simulink model "benchmark_model"  (R2021a)
settings: Solver=ode1  StartTime=0.0  StopTime=Tend  FixedStep=0.0001  MaxStep=0.1  MinStep=0.0001  AbsTol=0.01  EnableMultiTasking=on
undefined symbols (not defined in the file): A1, A2, AL, AM0, AREA, BORE, C_EGR, c_f, c_T, CAIR, cCO, cCO2, cH2, cH2O, cHC, cN2, CO, CO2, cO2, DEN0, DiscIntNeverNeededParam, EGR_dia, EGR_sk, EX_AREA, EX_M_AR, EXO, FD0, FOM, FR0, FR_C1, FR_C2, FR_C3, FR_C4, FR_C5, H2, H2O, HC, INC, INO, KET, Kex, Kh, MAS0, MCh, MHC, MN2, MO2, MOLcylT, N2, O2, PR0, R150, Rabs, SPEC, TBORE, Th_HC, Th_knock, THEX, THIN, TM0 ... (+9)
libraries: pid_lib x1
(part 2 of 6)

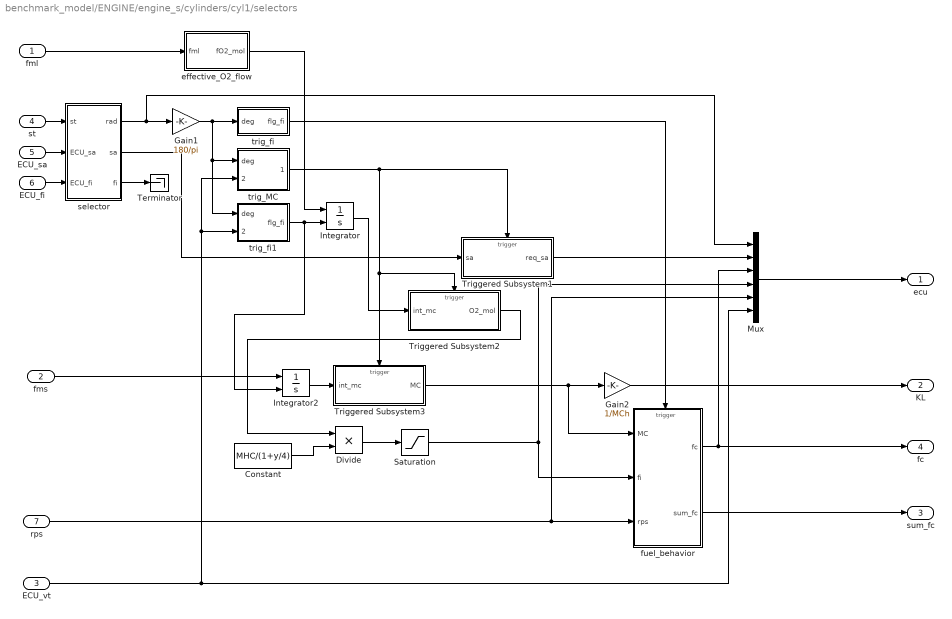
== system benchmark_model/ENGINE/engine_s/cylinders/cyl1/selectors ==
  fml : Inport
  fms : Inport  Port=2
  ECU_vt : Inport  Port=3
  st : Inport  Port=4
  ECU_sa : Inport  Port=5
  ECU_fi : Inport  Port=6
  rps : Inport  Port=7
  Constant : Constant  Value=MHC/(1+y/4)
  Divide : Product
  Gain1 : Gain  Gain=180/pi
  Gain2 : Gain  Gain=1/MCh
  Integrator : Integrator  ExternalReset=rising
  Integrator2 : Integrator  ExternalReset=rising
  Mux : Mux  Inputs=6
  Saturation : Saturate  UpperLimit=inf  LowerLimit=0
  Terminator : Terminator
  Triggered Subsystem1 : Subsystem  TreatAsAtomicUnit=on
  Triggered Subsystem2 : Subsystem  TreatAsAtomicUnit=on
  Triggered Subsystem3 : Subsystem  TreatAsAtomicUnit=on
  effective_O2_flow : Subsystem
  fuel_behavior : Subsystem  TreatAsAtomicUnit=on
  selector : Subsystem
  trig_MC : Subsystem
  trig_fi : Subsystem
  trig_fi1 : Subsystem
  ecu : Outport
  KL : Outport  Port=2
  sum_fc : Outport  Port=3
  fc : Outport  Port=4
  wires:
  Triggered Subsystem2/1(O2_mol) -> Divide/1
  Gain1/1 -> trig_fi/1(deg), trig_fi1/1(deg), trig_MC/1(deg)
  ECU_fi/1 -> selector/3(ECU_fi)
  ECU_sa/1 -> selector/2(ECU_sa)
  st/1 -> selector/1(st)
  trig_MC/1(flg_inc) -> Triggered Subsystem3/Trigger, Triggered Subsystem2/Trigger, Triggered Subsystem1/Trigger
  rps/1 -> Mux/5, fuel_behavior/3(rps)
  selector/1(rad) -> Gain1/1, Mux/1
  Mux/1 -> ecu/1
  trig_fi/1(flg_fi) -> fuel_behavior/Trigger
  selector/2(sa) -> Triggered Subsystem1/1(sa)
  Triggered Subsystem1/1(req_sa) -> Mux/2
  trig_fi1/1(flg_fi) -> Integrator/2, Integrator2/2
  Integrator/1 -> Triggered Subsystem2/1(int_mc)
  fuel_behavior/1(fc) -> fc/1, Mux/3
  selector/3(fi) -> Terminator/1
  Gain2/1 -> KL/1
  Divide/1 -> Saturation/1
  fml/1 -> effective_O2_flow/1(fml)
  effective_O2_flow/1(fO2_mol) -> Integrator/1
  Constant/1 -> Divide/2
  Saturation/1 -> fuel_behavior/2(fi), Mux/4
  Integrator2/1 -> Triggered Subsystem3/1(int_mc)
  Triggered Subsystem3/1(MC) -> Gain2/1, fuel_behavior/1(MC)
  fms/1 -> Integrator2/1
  ECU_vt/1 -> trig_MC/2(ECU_vvt), trig_fi1/2(ECU_vvt), Mux/6
  fuel_behavior/2(sum_fc) -> sum_fc/1

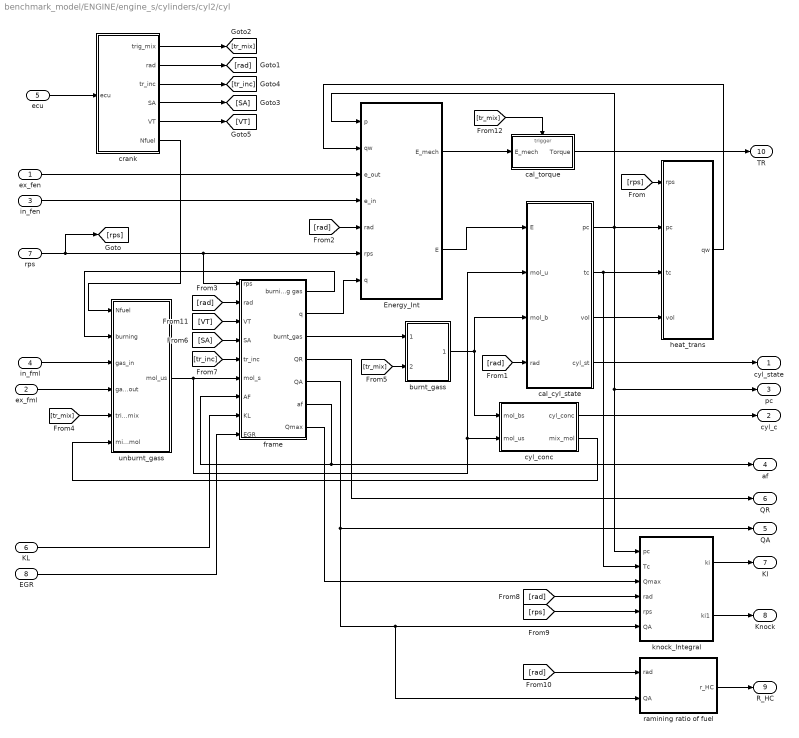
== system benchmark_model/ENGINE/engine_s/cylinders/cyl2/cyl ==
  ex_fen : Inport
  ex_fml : Inport  Port=2
  in_fen : Inport  Port=3
  in_fml : Inport  Port=4
  ecu : Inport  Port=5
  KL : Inport  Port=6
  rps : Inport  Port=7
  EGR : Inport  Port=8
  Energy_Int : Subsystem
  burnt_gass : Subsystem
  cal_cyl_state : Subsystem
  cal_torque : Subsystem
  crank : Subsystem
  cyl_conc : Subsystem
  frame : Subsystem
  heat_trans : Subsystem
  knock_Integral : Subsystem
  ramining ratio of fuel : Subsystem
  unburnt_gass : Subsystem
  cyl_state : Outport  InitialOutput=0
  cyl_c : Outport  Port=2  InitialOutput=0
  pc : Outport  Port=3  InitialOutput=0
  af : Outport  Port=4  InitialOutput=0
  QA : Outport  Port=5  InitialOutput=0
  QR : Outport  Port=6  InitialOutput=0
  KI : Outport  Port=7  InitialOutput=0
  Knock : Outport  Port=8  InitialOutput=0
  R_HC : Outport  Port=9  InitialOutput=0
  TR : Outport  Port=10  InitialOutput=0
  wires:
  [tr_mix] -> cal_torque/Trigger
  cal_torque/1(Torque) -> TR/1
  Energy_Int/1(E_mech) -> cal_torque/1(E_mech)
  crank/5(VT) -> [VT]
  [VT] -> frame/3(VT)
  frame/7(Qmax) -> knock_Integral/3(Qmax)
  ramining ratio of fuel/1(r_HC) -> R_HC/1
  [rad] -> ramining ratio of fuel/1(rad)
  knock_Integral/2(ki1) -> Knock/1
  [rps] -> knock_Integral/5(rps)
  frame/5(QA) -> knock_Integral/6(QA), ramining ratio of fuel/2(QA), QA/1
  [rad] -> knock_Integral/4(rad)
  EGR/1 -> frame/9(EGR)
  knock_Integral/1(ki) -> KI/1
  frame/4(QR) -> QR/1
  KL/1 -> frame/8(KL)
  [SA] -> frame/4(SA)
  crank/4(SA) -> [SA]
  Energy_Int/2(E) -> cal_cyl_state/1(E)
  cal_cyl_state/2(tc) -> heat_trans/3(tc), knock_Integral/2(Tc)
  cal_cyl_state/3(vol) -> heat_trans/4(vol)
  cal_cyl_state/4(cyl_st) -> cyl_state/1
  [rad] -> cal_cyl_state/4(rad)
  cal_cyl_state/1(pc) -> knock_Integral/1(pc), pc/1, Energy_Int/1(p), heat_trans/2(pc)
  crank/3(tr_inc) -> [tr_inc]
  cyl_conc/2(mix_mol) -> unburnt_gass/6(mix_mol)
  [tr_inc] -> frame/5(tr_inc)
  crank/6(Nfuel) -> unburnt_gass/1(Nfuel)
  frame/6(af) -> frame/7(AF), af/1
  crank/2(rad) -> [rad]
  [tr_mix] -> burnt_gass/2(tr_mix)
  [tr_mix] -> unburnt_gass/5(trig_mix)
  crank/1(trig_mix) -> [tr_mix]
  frame/1(burning gas) -> unburnt_gass/2(burning)
  ex_fml/1 -> unburnt_gass/4(gas_out)
  in_fen/1 -> Energy_Int/4(e_in)
  ex_fen/1 -> Energy_Int/3(e_out)
  [rad] -> frame/2(rad)
  [rad] -> Energy_Int/5(rad)
  ecu/1 -> crank/1(ecu)
  [rps] -> heat_trans/1(rps)
  cyl_conc/1(cyl_conc) -> cyl_c/1
  burnt_gass/1(mol_bs) -> cyl_conc/1(mol_bs), cal_cyl_state/3(mol_b)
  in_fml/1 -> unburnt_gass/3(gas_in)
  rps/1 -> Energy_Int/6(rps), frame/1(rps), [rps]
  unburnt_gass/1(mol_us) -> frame/6(mol_s), cal_cyl_state/2(mol_u), cyl_conc/2(mol_us)
  frame/3(burnt_gas) -> burnt_gass/1(gas_in)
  frame/2(q) -> Energy_Int/7(q)
  heat_trans/1(qw) -> Energy_Int/2(qw)

== system benchmark_model/ENGINE/engine_s/cylinders/cyl2/ex_valve ==
  d_st : Inport
  d_c : Inport  Port=2
  ecu : Inport  Port=3
  u_st : Inport  Port=4  PortDimensions=4
  u_c : Inport  Port=5
  Constant : Constant  Value=WOM
  Constant1 : Constant  Value=4*pi
  Gain : Gain  Gain=180/pi
  Lookup Table1 : Lookup  InputValues=THEX  Table=VAREX
  Math Function : Math  Operator=mod  SignedPower=on  SaturateOnIntegerOverflow=on
  Selector : Selector  InputPortWidth=6  IndexOptions=Index vector (dialog)  Indices=1  OutputSizes=[(-2)]
  cal_flow : MATLAB Function  TreatAsAtomicUnit=on
  fen : Outport  PortDimensions=1
  fml : Outport  Port=2  PortDimensions=7
  wires:
  Constant1/1 -> Math Function/2
  Selector/1 -> Math Function/1
  Math Function/1 -> Gain/1
  Gain/1 -> Lookup Table1/1
  Constant/1 -> cal_flow/6(WOM)
  cal_flow/2(fml) -> fml/1
  d_c/1 -> cal_flow/5(c_out)
  d_st/1 -> cal_flow/4(outlet)
  u_c/1 -> cal_flow/3(c_in)
  u_st/1 -> cal_flow/2(inlet)
  Lookup Table1/1 -> cal_flow/1(area)
  cal_flow/1(fen) -> fen/1
  ecu/1 -> Selector/1

== system benchmark_model/ENGINE/engine_s/cylinders/cyl2/in_valve ==
  d_c : Inport
  d_st : Inport  Port=2
  ecu : Inport  Port=3
  in_vt : Inport  Port=4
  u_st : Inport  Port=5
  u_c : Inport  Port=6
  Add : Sum  Inputs=-+
  Constant : Constant  Value=WOM
  Gain : Gain  Gain=180/pi
  Lookup Table : Lookup  InputValues=THIN  Table=VARIN
  Selector1 : Selector  InputPortWidth=6  IndexOptions=Index vector (dialog)  Indices=1  OutputSizes=[(-2)]
  cal_flow : MATLAB Function  TreatAsAtomicUnit=on
  fen : Outport  PortDimensions=1
  fml : Outport  Port=2  PortDimensions=7
  fms : Outport  Port=3  PortDimensions=1
  wires:
  Add/1 -> Gain/1
  Selector1/1 -> Add/2
  in_vt/1 -> Add/1
  Constant/1 -> cal_flow/6(WOM)
  cal_flow/3(fms) -> fms/1
  cal_flow/2(fml) -> fml/1
  d_c/1 -> cal_flow/5(c_out)
  u_c/1 -> cal_flow/3(c_in)
  cal_flow/1(fen) -> fen/1
  d_st/1 -> cal_flow/4(outlet)
  Lookup Table/1 -> cal_flow/1(area)
  u_st/1 -> cal_flow/2(inlet)
  ecu/1 -> Selector1/1
  Gain/1 -> Lookup Table/1

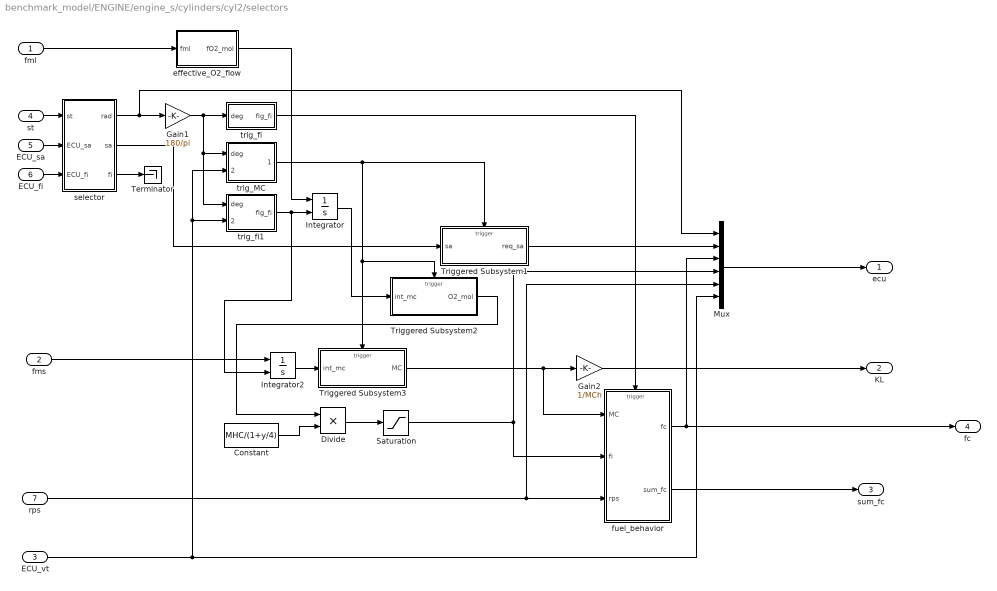
== system benchmark_model/ENGINE/engine_s/cylinders/cyl2/selectors ==
  fml : Inport
  fms : Inport  Port=2
  ECU_vt : Inport  Port=3
  st : Inport  Port=4
  ECU_sa : Inport  Port=5
  ECU_fi : Inport  Port=6
  rps : Inport  Port=7
  Constant : Constant  Value=MHC/(1+y/4)
  Divide : Product
  Gain1 : Gain  Gain=180/pi
  Gain2 : Gain  Gain=1/MCh
  Integrator : Integrator  ExternalReset=rising
  Integrator2 : Integrator  ExternalReset=rising
  Mux : Mux  Inputs=6
  Saturation : Saturate  UpperLimit=inf  LowerLimit=0
  Terminator : Terminator
  Triggered Subsystem1 : Subsystem  TreatAsAtomicUnit=on
  Triggered Subsystem2 : Subsystem  TreatAsAtomicUnit=on
  Triggered Subsystem3 : Subsystem  TreatAsAtomicUnit=on
  effective_O2_flow : Subsystem
  fuel_behavior : Subsystem  TreatAsAtomicUnit=on
  selector : Subsystem
  trig_MC : Subsystem
  trig_fi : Subsystem
  trig_fi1 : Subsystem
  ecu : Outport
  KL : Outport  Port=2
  sum_fc : Outport  Port=3
  fc : Outport  Port=4
  wires:
  fuel_behavior/2(sum_fc) -> sum_fc/1
  ECU_vt/1 -> Mux/6, trig_fi1/2(ECU_vvt), trig_MC/2(ECU_vvt)
  fms/1 -> Integrator2/1
  Triggered Subsystem3/1(MC) -> fuel_behavior/1(MC), Gain2/1
  Integrator2/1 -> Triggered Subsystem3/1(int_mc)
  Saturation/1 -> Mux/4, fuel_behavior/2(fi)
  Constant/1 -> Divide/2
  effective_O2_flow/1(fO2_mol) -> Integrator/1
  fml/1 -> effective_O2_flow/1(fml)
  Divide/1 -> Saturation/1
  Gain2/1 -> KL/1
  selector/3(fi) -> Terminator/1
  Integrator/1 -> Triggered Subsystem2/1(int_mc)
  trig_fi1/1(flg_fi) -> Integrator2/2, Integrator/2
  Triggered Subsystem1/1(req_sa) -> Mux/2
  selector/2(sa) -> Triggered Subsystem1/1(sa)
  trig_fi/1(flg_fi) -> fuel_behavior/Trigger
  Mux/1 -> ecu/1
  selector/1(rad) -> Mux/1, Gain1/1
  rps/1 -> fuel_behavior/3(rps), Mux/5
  trig_MC/1(flg_inc) -> Triggered Subsystem1/Trigger, Triggered Subsystem2/Trigger, Triggered Subsystem3/Trigger
  st/1 -> selector/1(st)
  ECU_sa/1 -> selector/2(ECU_sa)
  ECU_fi/1 -> selector/3(ECU_fi)
  Gain1/1 -> trig_MC/1(deg), trig_fi1/1(deg), trig_fi/1(deg)
  Triggered Subsystem2/1(O2_mol) -> Divide/1
  fuel_behavior/1(fc) -> fc/1, Mux/3

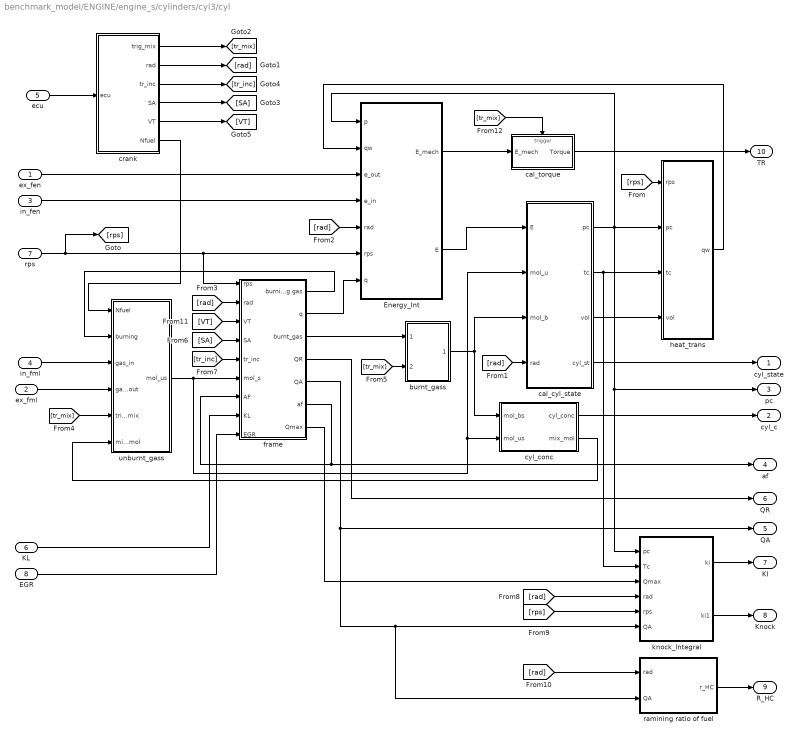
== system benchmark_model/ENGINE/engine_s/cylinders/cyl3/cyl ==
  ex_fen : Inport
  ex_fml : Inport  Port=2
  in_fen : Inport  Port=3
  in_fml : Inport  Port=4
  ecu : Inport  Port=5
  KL : Inport  Port=6
  rps : Inport  Port=7
  EGR : Inport  Port=8
  Energy_Int : Subsystem
  burnt_gass : Subsystem
  cal_cyl_state : Subsystem
  cal_torque : Subsystem
  crank : Subsystem
  cyl_conc : Subsystem
  frame : Subsystem
  heat_trans : Subsystem
  knock_Integral : Subsystem
  ramining ratio of fuel : Subsystem
  unburnt_gass : Subsystem
  cyl_state : Outport  InitialOutput=0
  cyl_c : Outport  Port=2  InitialOutput=0
  pc : Outport  Port=3  InitialOutput=0
  af : Outport  Port=4  InitialOutput=0
  QA : Outport  Port=5  InitialOutput=0
  QR : Outport  Port=6  InitialOutput=0
  KI : Outport  Port=7  InitialOutput=0
  Knock : Outport  Port=8  InitialOutput=0
  R_HC : Outport  Port=9  InitialOutput=0
  TR : Outport  Port=10  InitialOutput=0
  wires:
  heat_trans/1(qw) -> Energy_Int/2(qw)
  frame/2(q) -> Energy_Int/7(q)
  frame/3(burnt_gas) -> burnt_gass/1(gas_in)
  unburnt_gass/1(mol_us) -> cyl_conc/2(mol_us), cal_cyl_state/2(mol_u), frame/6(mol_s)
  rps/1 -> [rps], frame/1(rps), Energy_Int/6(rps)
  in_fml/1 -> unburnt_gass/3(gas_in)
  burnt_gass/1(mol_bs) -> cal_cyl_state/3(mol_b), cyl_conc/1(mol_bs)
  cyl_conc/1(cyl_conc) -> cyl_c/1
  [rps] -> heat_trans/1(rps)
  ecu/1 -> crank/1(ecu)
  [rad] -> Energy_Int/5(rad)
  [rad] -> frame/2(rad)
  ex_fen/1 -> Energy_Int/3(e_out)
  in_fen/1 -> Energy_Int/4(e_in)
  ex_fml/1 -> unburnt_gass/4(gas_out)
  frame/1(burning gas) -> unburnt_gass/2(burning)
  crank/1(trig_mix) -> [tr_mix]
  [tr_mix] -> unburnt_gass/5(trig_mix)
  [tr_mix] -> burnt_gass/2(tr_mix)
  crank/2(rad) -> [rad]
  frame/6(af) -> af/1, frame/7(AF)
  crank/6(Nfuel) -> unburnt_gass/1(Nfuel)
  [tr_inc] -> frame/5(tr_inc)
  cyl_conc/2(mix_mol) -> unburnt_gass/6(mix_mol)
  crank/3(tr_inc) -> [tr_inc]
  cal_cyl_state/1(pc) -> heat_trans/2(pc), Energy_Int/1(p), pc/1, knock_Integral/1(pc)
  [rad] -> cal_cyl_state/4(rad)
  cal_cyl_state/4(cyl_st) -> cyl_state/1
  cal_cyl_state/3(vol) -> heat_trans/4(vol)
  cal_cyl_state/2(tc) -> knock_Integral/2(Tc), heat_trans/3(tc)
  Energy_Int/2(E) -> cal_cyl_state/1(E)
  crank/4(SA) -> [SA]
  [SA] -> frame/4(SA)
  KL/1 -> frame/8(KL)
  frame/4(QR) -> QR/1
  knock_Integral/1(ki) -> KI/1
  EGR/1 -> frame/9(EGR)
  [rad] -> knock_Integral/4(rad)
  frame/5(QA) -> QA/1, ramining ratio of fuel/2(QA), knock_Integral/6(QA)
  [rps] -> knock_Integral/5(rps)
  knock_Integral/2(ki1) -> Knock/1
  [rad] -> ramining ratio of fuel/1(rad)
  ramining ratio of fuel/1(r_HC) -> R_HC/1
  frame/7(Qmax) -> knock_Integral/3(Qmax)
  [VT] -> frame/3(VT)
  crank/5(VT) -> [VT]
  Energy_Int/1(E_mech) -> cal_torque/1(E_mech)
  cal_torque/1(Torque) -> TR/1
  [tr_mix] -> cal_torque/Trigger

== system benchmark_model/ENGINE/engine_s/cylinders/cyl3/ex_valve ==
  d_st : Inport
  d_c : Inport  Port=2
  ecu : Inport  Port=3
  u_st : Inport  Port=4  PortDimensions=4
  u_c : Inport  Port=5
  Constant : Constant  Value=WOM
  Constant1 : Constant  Value=4*pi
  Gain : Gain  Gain=180/pi
  Lookup Table1 : Lookup  InputValues=THEX  Table=VAREX
  Math Function : Math  Operator=mod  SignedPower=on  SaturateOnIntegerOverflow=on
  Selector : Selector  InputPortWidth=6  IndexOptions=Index vector (dialog)  Indices=1  OutputSizes=[(-2)]
  cal_flow : MATLAB Function  TreatAsAtomicUnit=on
  fen : Outport  PortDimensions=1
  fml : Outport  Port=2  PortDimensions=7
  wires:
  ecu/1 -> Selector/1
  cal_flow/1(fen) -> fen/1
  Lookup Table1/1 -> cal_flow/1(area)
  u_st/1 -> cal_flow/2(inlet)
  u_c/1 -> cal_flow/3(c_in)
  d_st/1 -> cal_flow/4(outlet)
  d_c/1 -> cal_flow/5(c_out)
  cal_flow/2(fml) -> fml/1
  Constant/1 -> cal_flow/6(WOM)
  Gain/1 -> Lookup Table1/1
  Math Function/1 -> Gain/1
  Selector/1 -> Math Function/1
  Constant1/1 -> Math Function/2

== system benchmark_model/ENGINE/engine_s/cylinders/cyl3/in_valve ==
  d_c : Inport
  d_st : Inport  Port=2
  ecu : Inport  Port=3
  in_vt : Inport  Port=4
  u_st : Inport  Port=5
  u_c : Inport  Port=6
  Add : Sum  Inputs=-+
  Constant : Constant  Value=WOM
  Gain : Gain  Gain=180/pi
  Lookup Table : Lookup  InputValues=THIN  Table=VARIN
  Selector1 : Selector  InputPortWidth=6  IndexOptions=Index vector (dialog)  Indices=1  OutputSizes=[(-2)]
  cal_flow : MATLAB Function  TreatAsAtomicUnit=on
  fen : Outport  PortDimensions=1
  fml : Outport  Port=2  PortDimensions=7
  fms : Outport  Port=3  PortDimensions=1
  wires:
  Gain/1 -> Lookup Table/1
  ecu/1 -> Selector1/1
  u_st/1 -> cal_flow/2(inlet)
  Lookup Table/1 -> cal_flow/1(area)
  d_st/1 -> cal_flow/4(outlet)
  cal_flow/1(fen) -> fen/1
  u_c/1 -> cal_flow/3(c_in)
  d_c/1 -> cal_flow/5(c_out)
  cal_flow/2(fml) -> fml/1
  cal_flow/3(fms) -> fms/1
  Constant/1 -> cal_flow/6(WOM)
  in_vt/1 -> Add/1
  Selector1/1 -> Add/2
  Add/1 -> Gain/1

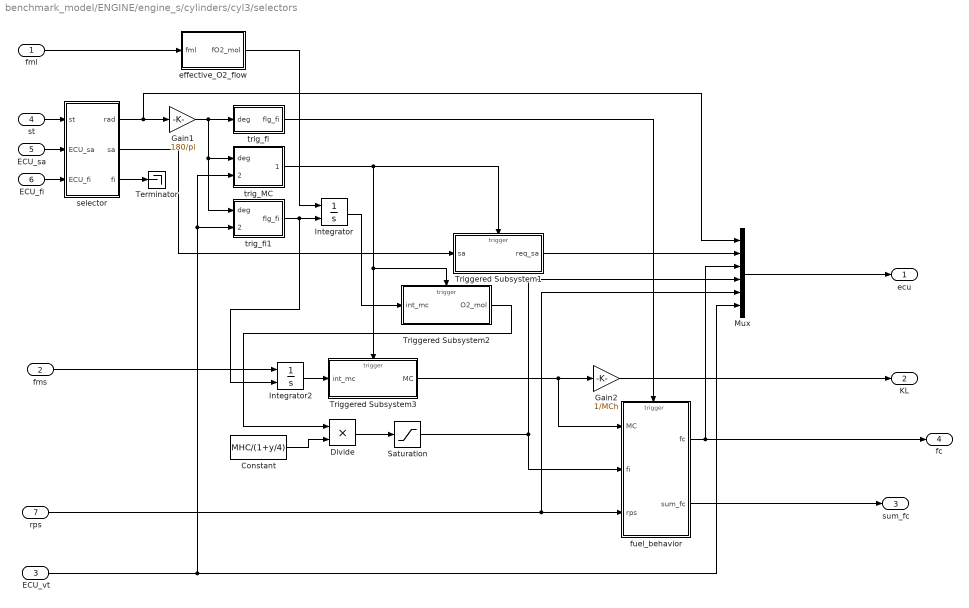
== system benchmark_model/ENGINE/engine_s/cylinders/cyl3/selectors ==
  fml : Inport
  fms : Inport  Port=2
  ECU_vt : Inport  Port=3
  st : Inport  Port=4
  ECU_sa : Inport  Port=5
  ECU_fi : Inport  Port=6
  rps : Inport  Port=7
  Constant : Constant  Value=MHC/(1+y/4)
  Divide : Product
  Gain1 : Gain  Gain=180/pi
  Gain2 : Gain  Gain=1/MCh
  Integrator : Integrator  ExternalReset=rising
  Integrator2 : Integrator  ExternalReset=rising
  Mux : Mux  Inputs=6
  Saturation : Saturate  UpperLimit=inf  LowerLimit=0
  Terminator : Terminator
  Triggered Subsystem1 : Subsystem  TreatAsAtomicUnit=on
  Triggered Subsystem2 : Subsystem  TreatAsAtomicUnit=on
  Triggered Subsystem3 : Subsystem  TreatAsAtomicUnit=on
  effective_O2_flow : Subsystem
  fuel_behavior : Subsystem  TreatAsAtomicUnit=on
  selector : Subsystem
  trig_MC : Subsystem
  trig_fi : Subsystem
  trig_fi1 : Subsystem
  ecu : Outport
  KL : Outport  Port=2
  sum_fc : Outport  Port=3
  fc : Outport  Port=4
  wires:
  Triggered Subsystem2/1(O2_mol) -> Divide/1
  Gain1/1 -> trig_fi/1(deg), trig_fi1/1(deg), trig_MC/1(deg)
  ECU_fi/1 -> selector/3(ECU_fi)
  ECU_sa/1 -> selector/2(ECU_sa)
  st/1 -> selector/1(st)
  trig_MC/1(flg_inc) -> Triggered Subsystem3/Trigger, Triggered Subsystem2/Trigger, Triggered Subsystem1/Trigger
  rps/1 -> Mux/5, fuel_behavior/3(rps)
  selector/1(rad) -> Gain1/1, Mux/1
  Mux/1 -> ecu/1
  trig_fi/1(flg_fi) -> fuel_behavior/Trigger
  selector/2(sa) -> Triggered Subsystem1/1(sa)
  Triggered Subsystem1/1(req_sa) -> Mux/2
  trig_fi1/1(flg_fi) -> Integrator/2, Integrator2/2
  Integrator/1 -> Triggered Subsystem2/1(int_mc)
  selector/3(fi) -> Terminator/1
  Gain2/1 -> KL/1
  Divide/1 -> Saturation/1
  fml/1 -> effective_O2_flow/1(fml)
  effective_O2_flow/1(fO2_mol) -> Integrator/1
  Constant/1 -> Divide/2
  Saturation/1 -> fuel_behavior/2(fi), Mux/4
  Integrator2/1 -> Triggered Subsystem3/1(int_mc)
  Triggered Subsystem3/1(MC) -> Gain2/1, fuel_behavior/1(MC)
  fms/1 -> Integrator2/1
  ECU_vt/1 -> trig_MC/2(ECU_vvt), trig_fi1/2(ECU_vvt), Mux/6
  fuel_behavior/2(sum_fc) -> sum_fc/1
  fuel_behavior/1(fc) -> fc/1, Mux/3

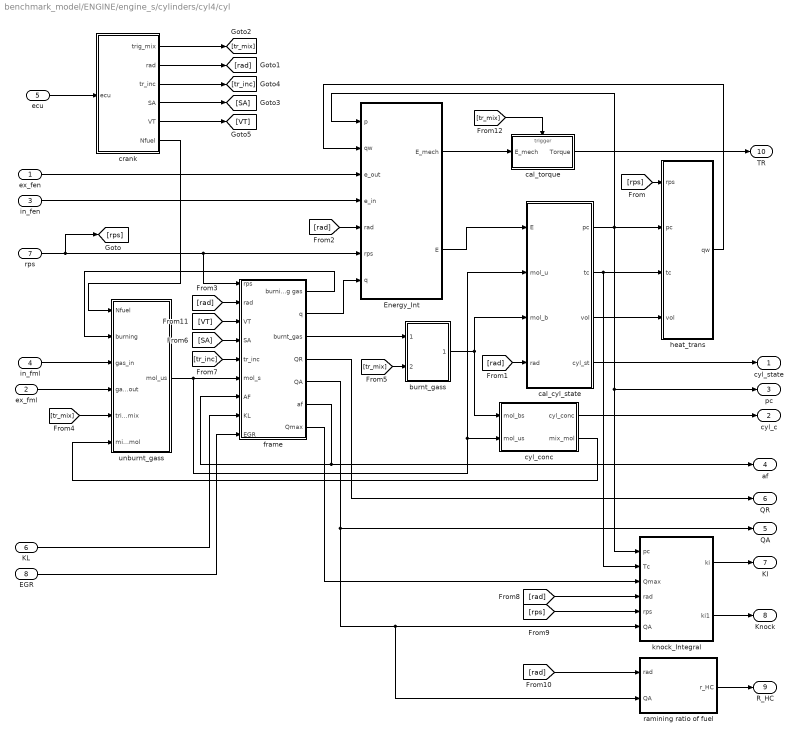
== system benchmark_model/ENGINE/engine_s/cylinders/cyl4/cyl ==
  ex_fen : Inport
  ex_fml : Inport  Port=2
  in_fen : Inport  Port=3
  in_fml : Inport  Port=4
  ecu : Inport  Port=5
  KL : Inport  Port=6
  rps : Inport  Port=7
  EGR : Inport  Port=8
  Energy_Int : Subsystem
  burnt_gass : Subsystem
  cal_cyl_state : Subsystem
  cal_torque : Subsystem
  crank : Subsystem
  cyl_conc : Subsystem
  frame : Subsystem
  heat_trans : Subsystem
  knock_Integral : Subsystem
  ramining ratio of fuel : Subsystem
  unburnt_gass : Subsystem
  cyl_state : Outport  InitialOutput=0
  cyl_c : Outport  Port=2  InitialOutput=0
  pc : Outport  Port=3  InitialOutput=0
  af : Outport  Port=4  InitialOutput=0
  QA : Outport  Port=5  InitialOutput=0
  QR : Outport  Port=6  InitialOutput=0
  KI : Outport  Port=7  InitialOutput=0
  Knock : Outport  Port=8  InitialOutput=0
  R_HC : Outport  Port=9  InitialOutput=0
  TR : Outport  Port=10  InitialOutput=0
  wires:
  [tr_mix] -> cal_torque/Trigger
  cal_torque/1(Torque) -> TR/1
  Energy_Int/1(E_mech) -> cal_torque/1(E_mech)
  crank/5(VT) -> [VT]
  [VT] -> frame/3(VT)
  frame/7(Qmax) -> knock_Integral/3(Qmax)
  ramining ratio of fuel/1(r_HC) -> R_HC/1
  [rad] -> ramining ratio of fuel/1(rad)
  knock_Integral/2(ki1) -> Knock/1
  [rps] -> knock_Integral/5(rps)
  frame/5(QA) -> knock_Integral/6(QA), ramining ratio of fuel/2(QA), QA/1
  [rad] -> knock_Integral/4(rad)
  EGR/1 -> frame/9(EGR)
  knock_Integral/1(ki) -> KI/1
  frame/4(QR) -> QR/1
  KL/1 -> frame/8(KL)
  [SA] -> frame/4(SA)
  crank/4(SA) -> [SA]
  Energy_Int/2(E) -> cal_cyl_state/1(E)
  cal_cyl_state/2(tc) -> heat_trans/3(tc), knock_Integral/2(Tc)
  cal_cyl_state/3(vol) -> heat_trans/4(vol)
  cal_cyl_state/4(cyl_st) -> cyl_state/1
  [rad] -> cal_cyl_state/4(rad)
  cal_cyl_state/1(pc) -> knock_Integral/1(pc), pc/1, Energy_Int/1(p), heat_trans/2(pc)
  crank/3(tr_inc) -> [tr_inc]
  cyl_conc/2(mix_mol) -> unburnt_gass/6(mix_mol)
  [tr_inc] -> frame/5(tr_inc)
  crank/6(Nfuel) -> unburnt_gass/1(Nfuel)
  frame/6(af) -> frame/7(AF), af/1
  crank/2(rad) -> [rad]
  [tr_mix] -> burnt_gass/2(tr_mix)
  [tr_mix] -> unburnt_gass/5(trig_mix)
  crank/1(trig_mix) -> [tr_mix]
  frame/1(burning gas) -> unburnt_gass/2(burning)
  ex_fml/1 -> unburnt_gass/4(gas_out)
  in_fen/1 -> Energy_Int/4(e_in)
  ex_fen/1 -> Energy_Int/3(e_out)
  [rad] -> frame/2(rad)
  [rad] -> Energy_Int/5(rad)
  ecu/1 -> crank/1(ecu)
  [rps] -> heat_trans/1(rps)
  cyl_conc/1(cyl_conc) -> cyl_c/1
  burnt_gass/1(mol_bs) -> cyl_conc/1(mol_bs), cal_cyl_state/3(mol_b)
  in_fml/1 -> unburnt_gass/3(gas_in)
  rps/1 -> Energy_Int/6(rps), frame/1(rps), [rps]
  unburnt_gass/1(mol_us) -> frame/6(mol_s), cal_cyl_state/2(mol_u), cyl_conc/2(mol_us)
  frame/3(burnt_gas) -> burnt_gass/1(gas_in)
  frame/2(q) -> Energy_Int/7(q)
  heat_trans/1(qw) -> Energy_Int/2(qw)

== system benchmark_model/ENGINE/engine_s/cylinders/cyl4/ex_valve ==
  d_st : Inport
  d_c : Inport  Port=2
  ecu : Inport  Port=3
  u_st : Inport  Port=4  PortDimensions=4
  u_c : Inport  Port=5
  Constant : Constant  Value=WOM
  Constant1 : Constant  Value=4*pi
  Gain : Gain  Gain=180/pi
  Lookup Table1 : Lookup  InputValues=THEX  Table=VAREX
  Math Function : Math  Operator=mod  SignedPower=on  SaturateOnIntegerOverflow=on
  Selector : Selector  InputPortWidth=6  IndexOptions=Index vector (dialog)  Indices=1  OutputSizes=[(-2)]
  cal_flow : MATLAB Function  TreatAsAtomicUnit=on
  fen : Outport  PortDimensions=1
  fml : Outport  Port=2  PortDimensions=7
  wires:
  Constant1/1 -> Math Function/2
  Selector/1 -> Math Function/1
  Math Function/1 -> Gain/1
  Gain/1 -> Lookup Table1/1
  Constant/1 -> cal_flow/6(WOM)
  cal_flow/2(fml) -> fml/1
  d_c/1 -> cal_flow/5(c_out)
  d_st/1 -> cal_flow/4(outlet)
  u_c/1 -> cal_flow/3(c_in)
  u_st/1 -> cal_flow/2(inlet)
  Lookup Table1/1 -> cal_flow/1(area)
  cal_flow/1(fen) -> fen/1
  ecu/1 -> Selector/1

== system benchmark_model/ENGINE/engine_s/cylinders/cyl4/in_valve ==
  d_c : Inport
  d_st : Inport  Port=2
  ecu : Inport  Port=3
  in_vt : Inport  Port=4
  u_st : Inport  Port=5
  u_c : Inport  Port=6
  Add : Sum  Inputs=-+
  Constant : Constant  Value=WOM
  Gain : Gain  Gain=180/pi
  Lookup Table : Lookup  InputValues=THIN  Table=VARIN
  Selector1 : Selector  InputPortWidth=6  IndexOptions=Index vector (dialog)  Indices=1  OutputSizes=[(-2)]
  cal_flow : MATLAB Function  TreatAsAtomicUnit=on
  fen : Outport  PortDimensions=1
  fml : Outport  Port=2  PortDimensions=7
  fms : Outport  Port=3  PortDimensions=1
  wires:
  Add/1 -> Gain/1
  Selector1/1 -> Add/2
  in_vt/1 -> Add/1
  Constant/1 -> cal_flow/6(WOM)
  cal_flow/3(fms) -> fms/1
  cal_flow/2(fml) -> fml/1
  d_c/1 -> cal_flow/5(c_out)
  u_c/1 -> cal_flow/3(c_in)
  cal_flow/1(fen) -> fen/1
  d_st/1 -> cal_flow/4(outlet)
  Lookup Table/1 -> cal_flow/1(area)
  u_st/1 -> cal_flow/2(inlet)
  ecu/1 -> Selector1/1
  Gain/1 -> Lookup Table/1

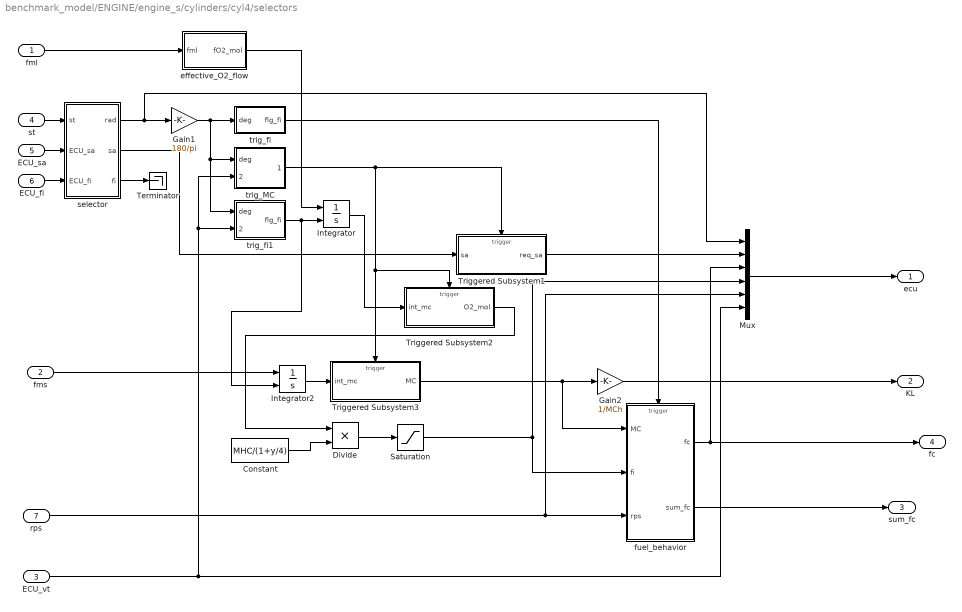
== system benchmark_model/ENGINE/engine_s/cylinders/cyl4/selectors ==
  fml : Inport
  fms : Inport  Port=2
  ECU_vt : Inport  Port=3
  st : Inport  Port=4
  ECU_sa : Inport  Port=5
  ECU_fi : Inport  Port=6
  rps : Inport  Port=7
  Constant : Constant  Value=MHC/(1+y/4)
  Divide : Product
  Gain1 : Gain  Gain=180/pi
  Gain2 : Gain  Gain=1/MCh
  Integrator : Integrator  ExternalReset=rising
  Integrator2 : Integrator  ExternalReset=rising
  Mux : Mux  Inputs=6
  Saturation : Saturate  UpperLimit=inf  LowerLimit=0
  Terminator : Terminator
  Triggered Subsystem1 : Subsystem  TreatAsAtomicUnit=on
  Triggered Subsystem2 : Subsystem  TreatAsAtomicUnit=on
  Triggered Subsystem3 : Subsystem  TreatAsAtomicUnit=on
  effective_O2_flow : Subsystem
  fuel_behavior : Subsystem  TreatAsAtomicUnit=on
  selector : Subsystem
  trig_MC : Subsystem
  trig_fi : Subsystem
  trig_fi1 : Subsystem
  ecu : Outport
  KL : Outport  Port=2
  sum_fc : Outport  Port=3
  fc : Outport  Port=4
  wires:
  fuel_behavior/2(sum_fc) -> sum_fc/1
  ECU_vt/1 -> Mux/6, trig_fi1/2(ECU_vvt), trig_MC/2(ECU_vvt)
  fms/1 -> Integrator2/1
  Triggered Subsystem3/1(MC) -> fuel_behavior/1(MC), Gain2/1
  Integrator2/1 -> Triggered Subsystem3/1(int_mc)
  Saturation/1 -> Mux/4, fuel_behavior/2(fi)
  Constant/1 -> Divide/2
  effective_O2_flow/1(fO2_mol) -> Integrator/1
  fml/1 -> effective_O2_flow/1(fml)
  Divide/1 -> Saturation/1
  Gain2/1 -> KL/1
  selector/3(fi) -> Terminator/1
  Integrator/1 -> Triggered Subsystem2/1(int_mc)
  trig_fi1/1(flg_fi) -> Integrator2/2, Integrator/2
  Triggered Subsystem1/1(req_sa) -> Mux/2
  selector/2(sa) -> Triggered Subsystem1/1(sa)
  trig_fi/1(flg_fi) -> fuel_behavior/Trigger
  Mux/1 -> ecu/1
  selector/1(rad) -> Mux/1, Gain1/1
  rps/1 -> fuel_behavior/3(rps), Mux/5
  trig_MC/1(flg_inc) -> Triggered Subsystem1/Trigger, Triggered Subsystem2/Trigger, Triggered Subsystem3/Trigger
  st/1 -> selector/1(st)
  ECU_sa/1 -> selector/2(ECU_sa)
  ECU_fi/1 -> selector/3(ECU_fi)
  Gain1/1 -> trig_MC/1(deg), trig_fi1/1(deg), trig_fi/1(deg)
  Triggered Subsystem2/1(O2_mol) -> Divide/1
  fuel_behavior/1(fc) -> fc/1, Mux/3

== system benchmark_model/ENGINE/engine_s/ex_chamber/In_vol/Enrgy_Int ==
  temp : Inport
  Enrgy_In : Inport  Port=2
  Enrgy_out : Inport  Port=3
  Enrgy_EGR : Inport  Port=4
  Constant1 : Constant  Value=TM0
  Gain : Gain  Gain=EX_M_AR*KET
  Sum : Sum  Inputs=-+--  InputSameDT=on  SaturateOnIntegerOverflow=on  OutDataTypeStr=Inherit: Same as first input
  Sum1 : Sum  Inputs=+-  InputSameDT=on  SaturateOnIntegerOverflow=on  OutDataTypeStr=Inherit: Same as first input
  energy_int : Integrator  InitialCondition=Einit
  E : Outport  InitialOutput=0
  wires:
  Gain/1 -> Sum/1
  Sum1/1 -> Gain/1
  Constant1/1 -> Sum1/2
  temp/1 -> Sum1/1
  Enrgy_In/1 -> Sum/2
  Enrgy_out/1 -> Sum/3
  Sum/1 -> energy_int/1
  energy_int/1 -> E/1
  Enrgy_EGR/1 -> Sum/4

== system benchmark_model/ENGINE/engine_s/ex_chamber/In_vol/Mol_Int ==
  nml_In : Inport
  nml_out : Inport  Port=2
  nml_EGR : Inport  Port=3
  Mol_Int : Integrator  InitialCondition=Ninit
  Sum : Sum  Inputs=+--  InputSameDT=on  SaturateOnIntegerOverflow=on  OutDataTypeStr=Inherit: Same as first input
  Nmol : Outport  InitialOutput=0
  wires:
  nml_In/1 -> Sum/1
  nml_out/1 -> Sum/2
  Sum/1 -> Mol_Int/1
  Mol_Int/1 -> Nmol/1
  nml_EGR/1 -> Sum/3

== system benchmark_model/ENGINE/engine_s/ex_chamber/In_vol/cal_cyl_state ==
  E : Inport
  Nml : Inport  Port=2
  Constant : Constant  Value=VL
  Divide : Product  Inputs=*/
  Dot Product : DotProduct  InputSameDT=on  OutDataTypeStr=Inherit: Inherit via internal rule
  Dot Product1 : DotProduct  InputSameDT=on  OutDataTypeStr=Inherit: Inherit via internal rule
  Sum of Elements : Sum  Inputs=+
  cal_state : Subsystem
  freedom : Constant  Value=FOM
  weight_mol : Constant  Value=WOM
  V_temp : Outport  InitialOutput=0
  V_st : Outport  Port=2  InitialOutput=0
  V_c : Outport  Port=3  InitialOutput=0
  wires:
  cal_state/2(ex_temp) -> V_temp/1
  Sum of Elements/1 -> cal_state/2(n), Divide/2
  freedom/1 -> Dot Product1/2
  Nml/1 -> Sum of Elements/1, Dot Product/2, Dot Product1/1, Divide/1
  weight_mol/1 -> Dot Product/1
  cal_state/1(ex_st) -> V_st/1
  Constant/1 -> cal_state/5(vol)
  E/1 -> cal_state/4(E)
  Divide/1 -> V_c/1
  Dot Product/1 -> cal_state/1(m)
  Dot Product1/1 -> cal_state/3(f)

== system benchmark_model/ENGINE/engine_s/in_chamber/In_vol/Enrgy_Int ==
  Enrgy_In : Inport
  Enrgy_out : Inport  Port=2
  Enrgy_EGR : Inport  Port=3
  Mass_Int : Integrator  InitialCondition=Einit
  Sum : Sum  Inputs=++-  InputSameDT=on  SaturateOnIntegerOverflow=on  OutDataTypeStr=Inherit: Same as first input
  X_dens : Outport  InitialOutput=0
  wires:
  Mass_Int/1 -> X_dens/1
  Sum/1 -> Mass_Int/1
  Enrgy_In/1 -> Sum/2
  Enrgy_out/1 -> Sum/3
  Enrgy_EGR/1 -> Sum/1

== system benchmark_model/ENGINE/engine_s/in_chamber/In_vol/Mol_Int ==
  nml_In : Inport
  nml_out : Inport  Port=2
  nml_EGR : Inport  Port=3
  Divide : Product  Inputs=/*
  Divide1 : Product  Inputs=*/
  Mol_Int : Integrator  InitialCondition=Ninit
  Sum : Sum  Inputs=++-  InputSameDT=on  SaturateOnIntegerOverflow=on  OutDataTypeStr=Inherit: Same as first input
  Sum of Elements : Sum  Inputs=+
  signiture_EGR : Subsystem
  signiture_EGR1 : Subsystem
  signiture_EGR2 : Subsystem
  signiture_EGR3 : Subsystem
  signiture_EGR4 : Subsystem
  Nmol : Outport  InitialOutput=0
  C_signed_C : Outport  Port=2  InitialOutput=0
  C_C : Outport  Port=3  InitialOutput=0
  wires:
  Sum/1 -> Mol_Int/1
  nml_In/1 -> signiture_EGR1/1(In)
  nml_out/1 -> signiture_EGR2/1(In)
  nml_EGR/1 -> signiture_EGR/1(In)
  signiture_EGR/1(Out) -> Sum/1
  signiture_EGR1/1(Out) -> Sum/2
  signiture_EGR2/1(Out) -> Sum/3
  Mol_Int/1 -> signiture_EGR3/1(In)
  signiture_EGR3/1(Out) -> Nmol/1, Sum of Elements/1, signiture_EGR4/1(In)
  Sum of Elements/1 -> Divide/1, Divide1/2
  signiture_EGR3/2(signed_C) -> Divide/2
  Divide/1 -> C_signed_C/1, signiture_EGR2/2(C_signed_C)
  Divide1/1 -> C_C/1
  signiture_EGR4/1(Out) -> Divide1/1

== system benchmark_model/ENGINE/engine_s/in_chamber/In_vol/cal_cyl_state ==
  E : Inport
  Nml : Inport  Port=2
  Constant : Constant  Value=VL
  Divide : Product  Inputs=*/
  Dot Product1 : DotProduct  InputSameDT=on  OutDataTypeStr=Inherit: Inherit via internal rule
  Dot Product2 : DotProduct  InputSameDT=on  OutDataTypeStr=Inherit: Inherit via internal rule
  Sum of Elements : Sum  Inputs=+
  cal_state : Subsystem
  freedom : Constant  Value=FOM
  weight_mol : Constant  Value=WOM
  V_st : Outport  InitialOutput=0
  V_c : Outport  Port=2  InitialOutput=0
  wires:
  Divide/1 -> V_c/1
  E/1 -> cal_state/4(E)
  Constant/1 -> cal_state/5(vol)
  cal_state/1(cyl_st) -> V_st/1
  Nml/1 -> Divide/1, Sum of Elements/1, Dot Product1/2, Dot Product2/1
  Sum of Elements/1 -> Divide/2, cal_state/2(n)
  Dot Product1/1 -> cal_state/1(m)
  weight_mol/1 -> Dot Product1/1
  Dot Product2/1 -> cal_state/3(f)
  freedom/1 -> Dot Product2/2

== system benchmark_model/ENGINE/engine_s/rpm_dynamics1/stroke/mod720(u,4*pi) ==
  u : Inport
  Constant7 : Constant  Value=4*pi
  Math Function : Math  Operator=mod  SignedPower=on  SaturateOnIntegerOverflow=on
  y : Outport
  wires:
  Constant7/1 -> Math Function/2
  u/1 -> Math Function/1
  Math Function/1 -> y/1

== system benchmark_model/ENGINE/engine_s/rpm_dynamics1/stroke/mod720(u,4*pi)1 ==
  u : Inport
  Constant7 : Constant  Value=4*pi
  Math Function : Math  Operator=mod  SignedPower=on  SaturateOnIntegerOverflow=on
  y : Outport
  wires:
  Math Function/1 -> y/1
  u/1 -> Math Function/1
  Constant7/1 -> Math Function/2

== system benchmark_model/ENGINE/engine_s/rpm_dynamics1/stroke/mod720(u,4*pi)2 ==
  u : Inport
  Constant7 : Constant  Value=4*pi
  Math Function : Math  Operator=mod  SignedPower=on  SaturateOnIntegerOverflow=on
  y : Outport
  wires:
  Constant7/1 -> Math Function/2
  u/1 -> Math Function/1
  Math Function/1 -> y/1

== system benchmark_model/ENGINE/engine_s/rpm_dynamics1/stroke/mod720(u,4*pi)3 ==
  u : Inport
  Constant7 : Constant  Value=4*pi
  Math Function : Math  Operator=mod  SignedPower=on  SaturateOnIntegerOverflow=on
  y : Outport
  wires:
  Math Function/1 -> y/1
  u/1 -> Math Function/1
  Constant7/1 -> Math Function/2

== system benchmark_model/ENGINE/engine_s/cylinders/cyl1/cyl/Energy_Int ==
  p : Inport
  qw : Inport  Port=2
  e_out : Inport  Port=3
  e_in : Inport  Port=4
  rad : Inport  Port=5
  rps : Inport  Port=6
  q : Inport  Port=7
  Constant : Constant  Value=PR0
  Product : Product  RndMeth=Zero
  Product1 : Product  RndMeth=Zero
  Subtract : Sum  Inputs=+-
  Sum2 : Sum  Inputs=+--+-  InputSameDT=on  SaturateOnIntegerOverflow=on  OutDataTypeStr=Inherit: Same as first input
  dvol : Subsystem
  int_e : Integrator  InitialCondition=(FD0/2.0)*PR0*VT
  int_pdv : Integrator
  E_mech : Outport  InitialOutput=0
  E : Outport  Port=2  InitialOutput=0
  wires:
  qw/1 -> Sum2/2
  e_out/1 -> Sum2/3
  Product/1 -> Sum2/5
  e_in/1 -> Sum2/4
  q/1 -> Sum2/1
  int_e/1 -> E/1
  Sum2/1 -> int_e/1
  rad/1 -> dvol/1(rad)
  dvol/1(dvol) -> Product1/1, Product/2
  rps/1 -> dvol/2(rps)
  int_pdv/1 -> E_mech/1
  p/1 -> Subtract/1, Product/1
  Constant/1 -> Subtract/2
  Subtract/1 -> Product1/2
  Product1/1 -> int_pdv/1

== system benchmark_model/ENGINE/engine_s/cylinders/cyl1/cyl/burnt_gass ==
  gas_in : Inport
  tr_mix : Inport  Port=2
  Mass_Int : Integrator  ExternalReset=rising  InitialCondition=[0;0;0;0;0;0;0]
  Memory2 : Memory
  mol_bs : Outport  PortDimensions=7  InitialOutput=0
  wires:
  Mass_Int/1 -> mol_bs/1
  gas_in/1 -> Mass_Int/1
  tr_mix/1 -> Memory2/1
  Memory2/1 -> Mass_Int/2

== system benchmark_model/ENGINE/engine_s/cylinders/cyl1/cyl/cal_cyl_state ==
  E : Inport
  mol_u : Inport  Port=2
  mol_b : Inport  Port=3
  rad : Inport  Port=4
  Add2 : Sum
  Constant : Constant  Value=SPEC
  Dot Product2 : DotProduct  InputSameDT=on  OutDataTypeStr=Inherit: Inherit via internal rule
  Dot Product3 : DotProduct  InputSameDT=on  OutDataTypeStr=Inherit: Inherit via internal rule
  Sum of Elements : Sum  Inputs=+
  cal_state : Subsystem
  cyl_vol : MATLAB Function  TreatAsAtomicUnit=on
  freedom : Constant  Value=FOM
  weight_mol : Constant  Value=WOM
  pc : Outport  InitialOutput=0
  tc : Outport  Port=2  InitialOutput=0
  vol : Outport  Port=3  InitialOutput=0
  cyl_st : Outport  Port=4  InitialOutput=0
  wires:
  E/1 -> cal_state/4(E)
  rad/1 -> cyl_vol/1(u)
  Constant/1 -> cyl_vol/2(SPEC)
  cal_state/1(pc) -> pc/1
  cal_state/2(tc) -> tc/1
  cal_state/3(cyl_st) -> cyl_st/1
  cyl_vol/1(vol) -> vol/1, cal_state/5(vol)
  weight_mol/1 -> Dot Product2/1
  mol_b/1 -> Add2/1
  mol_u/1 -> Add2/2
  Add2/1 -> Sum of Elements/1, Dot Product2/2, Dot Product3/1
  freedom/1 -> Dot Product3/2
  Sum of Elements/1 -> cal_state/2(n)
  Dot Product2/1 -> cal_state/1(m)
  Dot Product3/1 -> cal_state/3(f)

== system benchmark_model/ENGINE/engine_s/cylinders/cyl1/cyl/cal_torque ==
  E_mech : Inport
  Trigger : TriggerPort  VariantControl=(inherit)  PortDimensions=1
  Constant : Constant  Value=4*pi
  Divide : Product  Inputs=*/
  Subtract : Sum  Inputs=+-
  Unit Delay : UnitDelay  SampleTime=-1  HasFrameUpgradeWarning=on
  Torque : Outport
  wires:
  Unit Delay/1 -> Subtract/2
  E_mech/1 -> Subtract/1, Unit Delay/1
  Subtract/1 -> Divide/1
  Divide/1 -> Torque/1
  Constant/1 -> Divide/2

== system benchmark_model/ENGINE/engine_s/cylinders/cyl1/cyl/crank ==
  ecu : Inport
  Constant : Constant  Value=(180-EXO-1)*pi/180
  Constant2 : Constant  Value=(540+INC)*pi/180
  Relational Operator : RelationalOperator  OutDataTypeStr=boolean  RndMeth=Nearest
  Relational Operator2 : RelationalOperator  OutDataTypeStr=boolean  RndMeth=Nearest
  Selector : Selector  InputPortWidth=6  IndexOptions=Index vector (dialog)  Indices=1  OutputSizes=[(-2)]
  Selector1 : Selector  InputPortWidth=6  IndexOptions=Index vector (dialog)  Indices=[3]  OutputSizes=[(-2)]
  Selector2 : Selector  InputPortWidth=6  IndexOptions=Index vector (dialog)  Indices=[5]  OutputSizes=[(-2)]
  Selector3 : Selector  InputPortWidth=6  IndexOptions=Index vector (dialog)  Indices=2  OutputSizes=[(-2)]
  Selector4 : Selector  InputPortWidth=6  IndexOptions=Index vector (dialog)  Indices=6  OutputSizes=[(-2)]
  Selector5 : Selector  InputPortWidth=6  IndexOptions=Index vector (dialog)  Indices=6  OutputSizes=[(-2)]
  Subsystem1 : Subsystem
  Subtract : Sum  Inputs=+++
  inj_start : Subsystem
  mol_flow_rate : Subsystem
  trig_mix : Outport  PortDimensions=1
  rad : Outport  Port=2
  tr_inc : Outport  Port=3  PortDimensions=1
  SA : Outport  Port=4
  VT : Outport  Port=5
  Nfuel : Outport  Port=6
  wires:
  Selector/1 -> inj_start/1(rad), rad/1, Relational Operator2/1, Relational Operator/1
  Constant/1 -> Relational Operator/2
  ecu/1 -> Selector5/1, Selector4/1, Selector/1, Selector3/1, Selector2/1, Selector1/1
  Selector2/1 -> mol_flow_rate/1(rps)  "rps"
  Relational Operator2/1 -> tr_inc/1
  Selector3/1 -> SA/1
  Subtract/1 -> Relational Operator2/2
  Selector5/1 -> Subtract/1, VT/1
  Selector4/1 -> Subtract/3
  Constant2/1 -> Subtract/2
  Relational Operator/1 -> trig_mix/1
  inj_start/1(trig_inj) -> Subsystem1/1(trig_inj)
  Selector1/1 -> Subsystem1/2(fc)
  mol_flow_rate/1(N/s) -> Subsystem1/3(N/s)
  Subsystem1/1(N_fuel) -> Nfuel/1

== system benchmark_model/ENGINE/engine_s/cylinders/cyl1/cyl/cyl_conc ==
  mol_bs : Inport
  mol_us : Inport  Port=2
  Add : Sum
  Divide : Product  Inputs=*/
  Sum of Elements : Sum  Inputs=+
  cyl_conc : Outport  PortDimensions=7
  mix_mol : Outport  Port=2  PortDimensions=7
  wires:
  Add/1 -> Sum of Elements/1, Divide/1, mix_mol/1
  Sum of Elements/1 -> Divide/2
  mol_us/1 -> Add/2
  mol_bs/1 -> Add/1
  Divide/1 -> cyl_conc/1

== system benchmark_model/ENGINE/engine_s/cylinders/cyl1/cyl/frame ==
  rps : Inport
  rad : Inport  Port=2
  VT : Inport  Port=3
  SA : Inport  Port=4
  tr_inc : Inport  Port=5
  mol_s : Inport  Port=6
  AF : Inport  Port=7
  KL : Inport  Port=8
  EGR : Inport  Port=9
  Init_cyl_gas : Subsystem
  Product : Product  RndMeth=Zero
  Product1 : Product  RndMeth=Zero
  Product2 : Product  RndMeth=Zero
  ratio_burnt1 : Subsystem
  burning gas : Outport
  q : Outport  Port=2
  burnt_gas : Outport  Port=3
  QR : Outport  Port=4
  QA : Outport  Port=5
  af : Outport  Port=6
  Qmax : Outport  Port=7
  wires:
  Init_cyl_gas/3(b_comp) -> Product2/2
  Product2/1 -> burnt_gas/1
  Product1/1 -> q/1
  Init_cyl_gas/1(init_gas) -> Product/2
  Product/1 -> burning gas/1
  Init_cyl_gas/2(Qmax) -> Qmax/1, Product1/2
  ratio_burnt1/1(burnt_ratio) -> Product/1, Product2/1, Product1/1
  rps/1 -> ratio_burnt1/1(rps)
  rad/1 -> ratio_burnt1/2(rad)
  Init_cyl_gas/4(af) -> af/1
  mol_s/1 -> Init_cyl_gas/2(mol_s)
  tr_inc/1 -> Init_cyl_gas/1(tr_inc)
  AF/1 -> ratio_burnt1/3(AF)
  KL/1 -> ratio_burnt1/4(KL)
  SA/1 -> ratio_burnt1/5(SA)
  ratio_burnt1/2(QR) -> QR/1
  EGR/1 -> ratio_burnt1/6(EGR)
  ratio_burnt1/3(Q) -> QA/1
  VT/1 -> ratio_burnt1/7(VT)

== system benchmark_model/ENGINE/engine_s/cylinders/cyl1/cyl/heat_trans ==
  rps : Inport
  pc : Inport  Port=2
  tc : Inport  Port=3
  vol : Inport  Port=4
  Constant5 : Constant  Value=TW0
  Gain : Gain  Gain=Kh
  Product : Product  RndMeth=Zero
  cal_cyl_ar : Subsystem
  cal_qw : Subsystem
  cyl_wall : Subsystem
  qw : Outport
  wires:
  pc/1 -> cal_qw/1(pc)
  rps/1 -> cal_qw/2(rps)
  tc/1 -> cal_qw/3(Tg)
  cyl_wall/1(Tw) -> cal_qw/4(Tw)
  cal_qw/1(qw) -> Product/2
  Product/1 -> Gain/1
  Constant5/1 -> cyl_wall/2(Tw0)
  vol/1 -> cal_cyl_ar/1(vol)
  cal_cyl_ar/1(cyl_ar) -> Product/1
  Gain/1 -> cyl_wall/1(qw_v), qw/1

== system benchmark_model/ENGINE/engine_s/cylinders/cyl1/cyl/knock_Integral ==
  pc : Inport
  Tc : Inport  Port=2
  Qmax : Inport  Port=3
  rad : Inport  Port=4
  rps : Inport  Port=5
  QA : Inport  Port=6
  Constant : Constant
  Constant1 : Constant  Value=(180-EXO-3)*pi/180
  Constant2 : Constant
  Logical Operator : Logic  Operator=OR  AllPortsSameDT=off  OutDataTypeStr=boolean
  Product : Product
  Relational Operator : RelationalOperator  OutDataTypeStr=boolean  RndMeth=Nearest
  Relational Operator1 : RelationalOperator  OutDataTypeStr=boolean  RndMeth=Nearest
  Subsystem1 : Subsystem
  Switch : Switch  Threshold=0.5
  Triggered Subsystem : Subsystem  TreatAsAtomicUnit=on
  ki : Outport
  ki1 : Outport  Port=2
  wires:
  pc/1 -> Subsystem1/1(pc)
  rps/1 -> Subsystem1/2(rps)
  Tc/1 -> Subsystem1/3(Tc)
  rad/1 -> Relational Operator1/1, Subsystem1/4(rad)
  Subsystem1/1(ki) -> Relational Operator/1, ki/1
  Constant/1 -> Relational Operator/2
  Constant1/1 -> Relational Operator1/2
  Product/1 -> ki1/1
  Qmax/1 -> Product/2
  QA/1 -> Switch/1, Triggered Subsystem/2(QA)
  Relational Operator/1 -> Logical Operator/1
  Relational Operator1/1 -> Switch/2, Logical Operator/2
  Logical Operator/1 -> Triggered Subsystem/Trigger
  Switch/1 -> Triggered Subsystem/1(QA_max)
  Constant2/1 -> Switch/3
  Triggered Subsystem/1(AI_Q) -> Product/1

== system benchmark_model/ENGINE/engine_s/cylinders/cyl1/cyl/ramining ratio of fuel ==
  rad : Inport
  QA : Inport  Port=2
  Constant1 : Constant  Value=(180-EXO-3)*pi/180
  Memory : Memory
  Relational Operator1 : RelationalOperator  OutDataTypeStr=boolean  RndMeth=Nearest
  Triggered Subsystem : Subsystem  TreatAsAtomicUnit=on
  r_HC : Outport
  wires:
  Constant1/1 -> Relational Operator1/2
  Triggered Subsystem/1(AI_Q) -> r_HC/1
  QA/1 -> Memory/1
  rad/1 -> Relational Operator1/1
  Relational Operator1/1 -> Triggered Subsystem/Trigger
  Memory/1 -> Triggered Subsystem/1(QA)

== system benchmark_model/ENGINE/engine_s/cylinders/cyl1/cyl/unburnt_gass ==
  Nfuel : Inport
  burning : Inport  Port=2
  gas_in : Inport  Port=3
  gas_out : Inport  Port=4
  trig_mix : Inport  Port=5
  mix_mol : Inport  Port=6
  Mass_Int : Integrator  ExternalReset=rising  InitialConditionSource=external  InitialCondition=MAS0
  Memory1 : Memory
  Memory2 : Memory
  Sum : Sum  Inputs=+--  InputSameDT=on  SaturateOnIntegerOverflow=on  OutDataTypeStr=Inherit: Same as first input
  add_fuel1 : Subsystem
  init&trig : Subsystem  mask{NHC=cHC*MOLcylT, NCO2=cCO2*MOLcylT, NCO=cCO*MOLcylT, NO2=cO2*MOLcylT, NH2=cH2*MOLcylT, NH2O=cH2O*MOLcylT, NN2=cN2*MOLcylT}
      mask prompts: NHC "initial HC mol"; NCO2 "initial CO2 mol"; NCO "initial CO mol"; NO2 "initial O2 mol"; NH2 "initial H2 mol"; NH2O "initial H2O mol"; NN2 "initial N2 mol"
  mol_us : Outport  InitialOutput=0
  wires:
  gas_out/1 -> Sum/2
  Sum/1 -> Mass_Int/1
  burning/1 -> Sum/3
  Mass_Int/1 -> mol_us/1
  mix_mol/1 -> Memory1/1
  init&trig/1(init) -> Mass_Int/3
  gas_in/1 -> add_fuel1/2(mol)
  Nfuel/1 -> add_fuel1/1(Nfuel)
  add_fuel1/1(add_fuel) -> Sum/1
  Memory2/1 -> init&trig/1(trig), Mass_Int/2
  trig_mix/1 -> Memory2/1
  Memory1/1 -> init&trig/2(value)

== system benchmark_model/ENGINE/engine_s/cylinders/cyl1/selectors/Triggered Subsystem1 ==
  sa : Inport
  Trigger : TriggerPort  VariantControl=(inherit)
  req_sa : Outport  InitialOutput=[20]
  wires:
  sa/1 -> req_sa/1

== system benchmark_model/ENGINE/engine_s/cylinders/cyl1/selectors/Triggered Subsystem2 ==
  int_mc : Inport
  Trigger : TriggerPort  VariantControl=(inherit)
  O2_mol : Outport  InitialOutput=[1.0e-19]
  wires:
  int_mc/1 -> O2_mol/1

== system benchmark_model/ENGINE/engine_s/cylinders/cyl1/selectors/Triggered Subsystem3 ==
  int_mc : Inport
  Trigger : TriggerPort  VariantControl=(inherit)
  MC : Outport  InitialOutput=[1.0e-19]
  wires:
  int_mc/1 -> MC/1

== system benchmark_model/ENGINE/engine_s/cylinders/cyl1/selectors/effective_O2_flow ==
  fml : Inport
  Gain : Gain  Gain=1+y/4
  Gain1 : Gain  Gain=0.5
  Gain2 : Gain  Gain=0.5
  Selector : Selector  InputPortWidth=7  IndexOptions=Index vector (dialog)  Indices=[4]  OutputSizes=1
  Selector1 : Selector  InputPortWidth=7  IndexOptions=Index vector (dialog)  Indices=[1]  OutputSizes=1
  Selector2 : Selector  InputPortWidth=7  IndexOptions=Index vector (dialog)  Indices=[3]  OutputSizes=1
  Selector3 : Selector  InputPortWidth=7  IndexOptions=Index vector (dialog)  Indices=[5]  OutputSizes=1
  Subtract : Sum  Inputs=+---
  fO2_mol : Outport
  wires:
  Subtract/1 -> fO2_mol/1
  fml/1 -> Selector/1, Selector1/1, Selector2/1, Selector3/1
  Selector/1 -> Subtract/1
  Selector1/1 -> Gain/1
  Gain/1 -> Subtract/2
  Selector2/1 -> Gain1/1
  Selector3/1 -> Gain2/1
  Gain1/1 -> Subtract/3
  Gain2/1 -> Subtract/4

== system benchmark_model/ENGINE/engine_s/cylinders/cyl1/selectors/fuel_behavior ==
  MC : Inport
  fi : Inport  Port=2
  rps : Inport  Port=3
  Trigger : TriggerPort  VariantControl=(inherit)
  Discrete-Time Integrator : DiscreteIntegrator  SampleTime=-1  ICPrevOutput=DiscIntNeverNeededParam  ICPrevScaledInput=DiscIntNeverNeededParam
  Terminator : Terminator
  Terminator3 : Terminator
  fc : Outport  InitialOutput=[0]
  sum_fc : Outport  Port=2  InitialOutput=[0]
  wires:
  fi/1 -> Discrete-Time Integrator/1, fc/1
  MC/1 -> Terminator3/1
  rps/1 -> Terminator/1
  Discrete-Time Integrator/1 -> sum_fc/1

== system benchmark_model/ENGINE/engine_s/cylinders/cyl1/selectors/selector ==
  st : Inport
  ECU_sa : Inport  Port=2
  ECU_fi : Inport  Port=3
  Saturation : Saturate  UpperLimit=inf  LowerLimit=0
  Selector : Selector  InputPortWidth=4  IndexOptions=Index vector (dialog)  Indices=[1]  OutputSizes=[(-2)]
  Selector2 : Selector  InputPortWidth=4  IndexOptions=Index vector (dialog)  Indices=[1]  OutputSizes=[(-2)]
  mod720(u,4*pi) : Subsystem
  rad : Outport
  sa : Outport  Port=2
  fi : Outport  Port=3
  wires:
  Selector/1 -> mod720(u,4*pi)/1(u)
  Saturation/1 -> fi/1
  mod720(u,4*pi)/1(y) -> rad/1
  st/1 -> Selector/1
  ECU_sa/1 -> Selector2/1
  ECU_fi/1 -> Saturation/1
  Selector2/1 -> sa/1

== system benchmark_model/ENGINE/engine_s/cylinders/cyl1/selectors/trig_MC ==
  deg : Inport
  ECU_vvt : Inport  Port=2
  Constant : Constant  Value=541+INC
  Gain : Gain  Gain=180/pi
  Relational Operator : RelationalOperator  OutDataTypeStr=boolean  RndMeth=Nearest
  Subtract : Sum
  flg_inc : Outport
  wires:
  deg/1 -> Relational Operator/1
  Relational Operator/1 -> flg_inc/1
  Subtract/1 -> Relational Operator/2
  ECU_vvt/1 -> Gain/1
  Constant/1 -> Subtract/2
  Gain/1 -> Subtract/1

== system benchmark_model/ENGINE/engine_s/cylinders/cyl1/selectors/trig_fi ==
  deg : Inport
  Constant : Constant  Value=361
  Relational Operator : RelationalOperator  OutDataTypeStr=boolean  RndMeth=Nearest
  flg_fi : Outport
  wires:
  Constant/1 -> Relational Operator/2
  deg/1 -> Relational Operator/1
  Relational Operator/1 -> flg_fi/1

== system benchmark_model/ENGINE/engine_s/cylinders/cyl1/selectors/trig_fi1 ==
  deg : Inport
  ECU_vvt : Inport  Port=2
  Constant : Constant  Value=360-INO-1
  Gain : Gain  Gain=180/pi
  Relational Operator : RelationalOperator  OutDataTypeStr=boolean  RndMeth=Nearest
  Subtract : Sum
  flg_fi : Outport
  wires:
  Relational Operator/1 -> flg_fi/1
  deg/1 -> Relational Operator/1
  ECU_vvt/1 -> Gain/1
  Gain/1 -> Subtract/1
  Subtract/1 -> Relational Operator/2
  Constant/1 -> Subtract/2

== system benchmark_model/ENGINE/engine_s/cylinders/cyl2/cyl/Energy_Int ==
  p : Inport
  qw : Inport  Port=2
  e_out : Inport  Port=3
  e_in : Inport  Port=4
  rad : Inport  Port=5
  rps : Inport  Port=6
  q : Inport  Port=7
  Constant : Constant  Value=PR0
  Product : Product  RndMeth=Zero
  Product1 : Product  RndMeth=Zero
  Subtract : Sum  Inputs=+-
  Sum2 : Sum  Inputs=+--+-  InputSameDT=on  SaturateOnIntegerOverflow=on  OutDataTypeStr=Inherit: Same as first input
  dvol : Subsystem
  int_e : Integrator  InitialCondition=(FD0/2.0)*PR0*VT
  int_pdv : Integrator
  E_mech : Outport  InitialOutput=0
  E : Outport  Port=2  InitialOutput=0
  wires:
  Product1/1 -> int_pdv/1
  Subtract/1 -> Product1/2
  Constant/1 -> Subtract/2
  p/1 -> Product/1, Subtract/1
  int_pdv/1 -> E_mech/1
  rps/1 -> dvol/2(rps)
  dvol/1(dvol) -> Product/2, Product1/1
  rad/1 -> dvol/1(rad)
  Sum2/1 -> int_e/1
  int_e/1 -> E/1
  q/1 -> Sum2/1
  e_in/1 -> Sum2/4
  Product/1 -> Sum2/5
  e_out/1 -> Sum2/3
  qw/1 -> Sum2/2

== system benchmark_model/ENGINE/engine_s/cylinders/cyl2/cyl/burnt_gass ==
  gas_in : Inport
  tr_mix : Inport  Port=2
  Mass_Int : Integrator  ExternalReset=rising  InitialCondition=[0;0;0;0;0;0;0]
  Memory2 : Memory
  mol_bs : Outport  PortDimensions=7  InitialOutput=0
  wires:
  Memory2/1 -> Mass_Int/2
  tr_mix/1 -> Memory2/1
  gas_in/1 -> Mass_Int/1
  Mass_Int/1 -> mol_bs/1

== system benchmark_model/ENGINE/engine_s/cylinders/cyl2/cyl/cal_cyl_state ==
  E : Inport
  mol_u : Inport  Port=2
  mol_b : Inport  Port=3
  rad : Inport  Port=4
  Add2 : Sum
  Constant : Constant  Value=SPEC
  Dot Product2 : DotProduct  InputSameDT=on  OutDataTypeStr=Inherit: Inherit via internal rule
  Dot Product3 : DotProduct  InputSameDT=on  OutDataTypeStr=Inherit: Inherit via internal rule
  Sum of Elements : Sum  Inputs=+
  cal_state : Subsystem
  cyl_vol : MATLAB Function  TreatAsAtomicUnit=on
  freedom : Constant  Value=FOM
  weight_mol : Constant  Value=WOM
  pc : Outport  InitialOutput=0
  tc : Outport  Port=2  InitialOutput=0
  vol : Outport  Port=3  InitialOutput=0
  cyl_st : Outport  Port=4  InitialOutput=0
  wires:
  Dot Product3/1 -> cal_state/3(f)
  Dot Product2/1 -> cal_state/1(m)
  Sum of Elements/1 -> cal_state/2(n)
  freedom/1 -> Dot Product3/2
  Add2/1 -> Dot Product3/1, Dot Product2/2, Sum of Elements/1
  mol_u/1 -> Add2/2
  mol_b/1 -> Add2/1
  weight_mol/1 -> Dot Product2/1
  cyl_vol/1(vol) -> cal_state/5(vol), vol/1
  cal_state/3(cyl_st) -> cyl_st/1
  cal_state/2(tc) -> tc/1
  cal_state/1(pc) -> pc/1
  Constant/1 -> cyl_vol/2(SPEC)
  rad/1 -> cyl_vol/1(u)
  E/1 -> cal_state/4(E)

== system benchmark_model/ENGINE/engine_s/cylinders/cyl2/cyl/cal_torque ==
  E_mech : Inport
  Trigger : TriggerPort  VariantControl=(inherit)  PortDimensions=1
  Constant : Constant  Value=4*pi
  Divide : Product  Inputs=*/
  Subtract : Sum  Inputs=+-
  Unit Delay : UnitDelay  SampleTime=-1  HasFrameUpgradeWarning=on
  Torque : Outport
  wires:
  Constant/1 -> Divide/2
  Divide/1 -> Torque/1
  Subtract/1 -> Divide/1
  E_mech/1 -> Unit Delay/1, Subtract/1
  Unit Delay/1 -> Subtract/2

== system benchmark_model/ENGINE/engine_s/cylinders/cyl2/cyl/crank ==
  ecu : Inport
  Constant : Constant  Value=(180-EXO-1)*pi/180
  Constant2 : Constant  Value=(540+INC)*pi/180
  Relational Operator : RelationalOperator  OutDataTypeStr=boolean  RndMeth=Nearest
  Relational Operator2 : RelationalOperator  OutDataTypeStr=boolean  RndMeth=Nearest
  Selector : Selector  InputPortWidth=6  IndexOptions=Index vector (dialog)  Indices=1  OutputSizes=[(-2)]
  Selector1 : Selector  InputPortWidth=6  IndexOptions=Index vector (dialog)  Indices=[3]  OutputSizes=[(-2)]
  Selector2 : Selector  InputPortWidth=6  IndexOptions=Index vector (dialog)  Indices=[5]  OutputSizes=[(-2)]
  Selector3 : Selector  InputPortWidth=6  IndexOptions=Index vector (dialog)  Indices=2  OutputSizes=[(-2)]
  Selector4 : Selector  InputPortWidth=6  IndexOptions=Index vector (dialog)  Indices=6  OutputSizes=[(-2)]
  Selector5 : Selector  InputPortWidth=6  IndexOptions=Index vector (dialog)  Indices=6  OutputSizes=[(-2)]
  Subsystem1 : Subsystem
  Subtract : Sum  Inputs=+++
  inj_start : Subsystem
  mol_flow_rate : Subsystem
  trig_mix : Outport  PortDimensions=1
  rad : Outport  Port=2
  tr_inc : Outport  Port=3  PortDimensions=1
  SA : Outport  Port=4
  VT : Outport  Port=5
  Nfuel : Outport  Port=6
  wires:
  Subsystem1/1(N_fuel) -> Nfuel/1
  mol_flow_rate/1(N/s) -> Subsystem1/3(N/s)
  Selector1/1 -> Subsystem1/2(fc)
  inj_start/1(trig_inj) -> Subsystem1/1(trig_inj)
  Relational Operator/1 -> trig_mix/1
  Constant2/1 -> Subtract/2
  Selector4/1 -> Subtract/3
  Selector5/1 -> VT/1, Subtract/1
  Subtract/1 -> Relational Operator2/2
  Selector3/1 -> SA/1
  Relational Operator2/1 -> tr_inc/1
  Selector2/1 -> mol_flow_rate/1(rps)  "rps"
  ecu/1 -> Selector1/1, Selector2/1, Selector3/1, Selector/1, Selector4/1, Selector5/1
  Constant/1 -> Relational Operator/2
  Selector/1 -> Relational Operator/1, Relational Operator2/1, rad/1, inj_start/1(rad)
